simulink model "mavsim_L_t"  (R2023b)
settings: Solver=ode45  StartTime=0.0  StopTime=40  RelTol=1e-3  EnableMultiTasking=on
values from neighbouring files (symbols this model uses):
  P = (eye(17) - L*H)*P    [Estimator.m]
undefined symbols (not defined in the file or in its folder): barometer, drawAircraft_v2, Euler_to_Ra2b, forces_moments, gps, plotmavstatevariables, POS_smoother2, Pressure2Altitude
libraries: simulink x4, spsStairGeneratorLib x3, shared6dof x1, aerolibnav x1
settings Model: Creator=beard  LastModifiedBy=13995
settings SolverCC: AlgebraicLoopSolver=TrustRegion
settings DataIOCC: SaveFormat=Array
settings OptimizationCC: ExpressionDepthLimit=2147483647  InitFltsAndDblsToZero=on  LifeSpan=inf
settings DebuggingCC: UnderspecifiedInitializationDetection=Classic  MergeDetectMultiDrivingBlocksExec=none  SolverPrmCheckMsg=warning  UnconnectedInputMsg=warning  UnconnectedOutputMsg=warning  UnconnectedLineMsg=warning  StateNameClashWarn=warning  SFUnexpectedBacktrackingDiag=warning  SFNoUnconditionalDefaultTransitionDiag=warning  SFExecutionAtInitializationDiag=none  ArithmeticOperatorsInVariantConditions=warning
settings HardwareCC: ProdBitPerPointer=32  ProdBitPerSizeT=32  ProdBitPerPtrDiffT=32  ProdLargestAtomicFloat=None  ProdIntDivRoundTo=Undefined  ProdEndianess=Unspecified  ProdWordSize=32  ProdHWDeviceType=32-bit Generic
settings ModelReferenceCC: EnableRefExpFcnMdlSchedulingChecks=on  PropagateSignalLabelsOutOfModel=off
settings SFSimCC: SimUseLocalCustomCode=off  CustomCodeUndefinedFunction=UseInterfaceOnly
settings RTWCC: RTWUseLocalCustomCode=off
settings CodeAppCC: StateflowObjectComments=on
settings GRTTargetCC: TargetLangStandard=C89/C90 (ANSI)  CombineOutputUpdateFcns=off  GRTInterface=on
settings ConfigComp: CovMetricSettings=dw  CovSaveCumulativeToWorkspaceVar=on  CovSaveSingleToWorkspaceVar=on  CovExternalEMLEnable=off  CovSFcnEnable=off
settings SimscapeCC: SimscapeNormalizeSystem=off

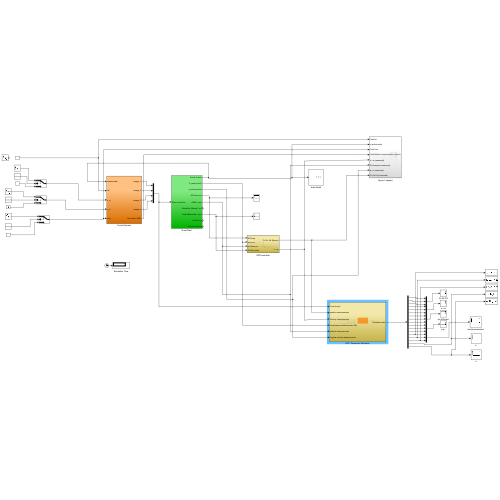
[thumbnail: Simulink's stored preview of the top-level diagram]
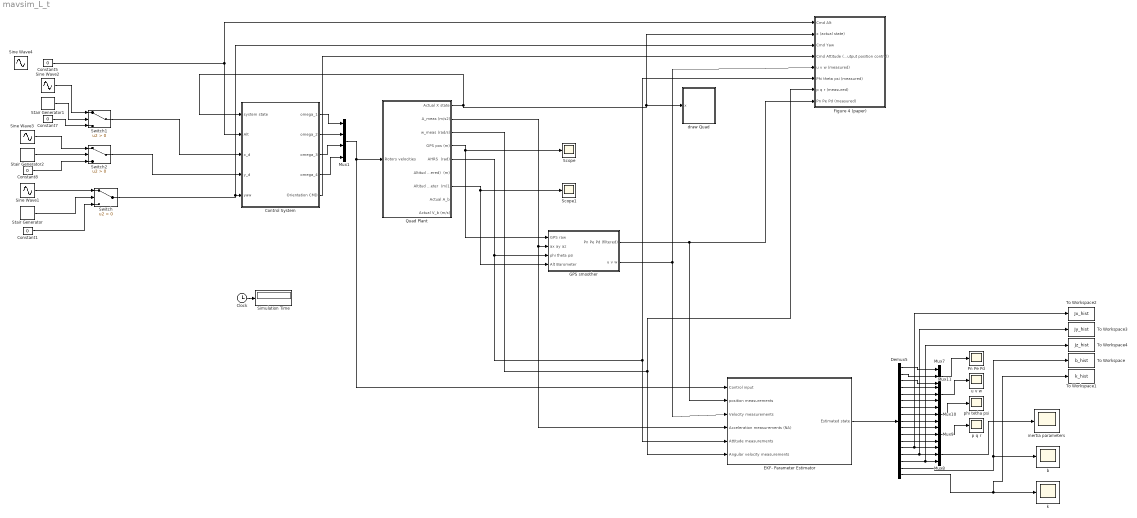
== system mavsim_L_t ==
  Clock : Clock
  Constant{1,5,7..8} (4 alike) : Constant  Value=0
  Control System : Subsystem
  Demux5 : Demux  Outputs=17
  EKF- Parameter Estimator : Subsystem
  Figure 4 (paper) : Subsystem
  GPS smoother : Subsystem
  Mux1 : Mux
  Mux{7..11} (5 alike) : Mux  Inputs=3
  Pn Pe Pd : Scope
  Quad Plant : Subsystem
  Scope : Scope
  Scope1 : Scope
  Simulation Time : Display
  Sine Wave1 : Sin  Amplitude=.45  Frequency=1.5  SampleTime=0
  Sine Wave2 : Sin  Frequency=2  SampleTime=0
  Sine Wave3 : Sin  Frequency=2  Phase=pi/2  SampleTime=0
  Sine Wave4 : Sin  Frequency=2  SampleTime=0
  Stair Generator : spsStairGeneratorLib/Stair Generator  t=[0, 5, 10, 15, 20, 25, 30 ,35,40]  e=[1, 1,1, 1,1,1,1,1,1]  Ts=0
  Stair Generator1 : spsStairGeneratorLib/Stair Generator  t=[0, 5, 10, 15, 20, 25, 30 ,35]  e="[1, 1,  1, 1, 1, 1, 1, 1]"  Ts=0
  Stair Generator2 : spsStairGeneratorLib/Stair Generator  t=[0, 5, 10, 15, 20, 25, 30 ,35]  e="[1, 1, 1 , 1, 1, 1, 1,  1]"  Ts=0
  Switch : Switch  Criteria=u2 > Threshold  SaturateOnIntegerOverflow=off  InputSameDT=off
  Switch1 : Switch  Criteria=u2 > Threshold  SaturateOnIntegerOverflow=off  InputSameDT=off
  Switch2 : Switch  Criteria=u2 > Threshold  SaturateOnIntegerOverflow=off  InputSameDT=off
  To Workspace : ToWorkspace  VariableName=b_hist  SaveFormat=Timeseries  SampleTime=-1
  To Workspace1 : ToWorkspace  VariableName=k_hist  SaveFormat=Timeseries  SampleTime=-1
  To Workspace2 : ToWorkspace  VariableName=Jx_hist  SaveFormat=Timeseries  SampleTime=-1
  To Workspace3 : ToWorkspace  VariableName=Jy_hist  SaveFormat=Timeseries  SampleTime=-1
  To Workspace4 : ToWorkspace  VariableName=Jz_hist  SaveFormat=Timeseries  SampleTime=-1
  b : Scope
  draw Quad : Subsystem
      mask init:
      | % parameters for drawing aircraft
      |   % scale size
      |   size = 20;
      |   fuse_l1    = 7;
      |   fuse_l2    = 4;
      |   fuse_l3    = 15;
      |   fuse_w     = 2;
      |   wing_l     = 6;
      |   wing_w     = 20;
      |   tail_l     = 3;
      |   tail_h     = 3;
      |   tailwing_w = 10;
      |   tailwing_l = 3;
      |   % colors
      |   red     = [1, 0, 0];
      |   green   = [0, 1, 0];
      |   blue    = [0, 0, 1];
      |   yellow  = [1,1,0];
      |   magenta = [0, 1, 1];
      |   
      | 
      | % define vertices and faces for aircraft
      |   V = [...
      |     fuse_l1,             0,             0;...        % point 1
      |     fuse_l2,            -fuse_w/2,     -fuse_w/2;... % point 2     
      |     fuse_l2,             fuse_w/2,     -fuse_w/2;... % point 3     
      |     fuse_l2,             fuse_w/2,      fuse_w/2;... % point 4
      |     fuse_l2,            -fuse_w/2,      fuse_w/2;... % point 5
      |    -fuse_l3,             0,             0;...        % point 6
      |     0,                   wing_w/2,      0;...        % point 7
      |    -wing_l,              wing_w/2,      0;...        % point 8
      |    -wing_l,             -wing_w/2,      0;...        % point 9
      |     0,                  -wing_w/2,      0;...        % point 10
      |    -fuse_l3+tailwing_l,  tailwing_w/2,  0;...        % point 11
      |    -fuse_l3,             tailwing_w/2,  0;...        % point 12
      |    -fuse_l3,            -tailwing_w/2,  0;...        % point 13
      |    -fuse_l3+tailwing_l, -tailwing_w/2,  0;...        % point 14
      |    -fuse_l3+tailwing_l,  0,             0;...        % point 15
      |    -fuse_l3+tailwing_l,  0,             -tail_h;...  % point 16
      |    -fuse_l3,             0,             -tail_h;...  % point 17
      |   ];
      |   
      |   F = [...
      |         1,  2,  3,  1;... % nose-top
      |         1,  3,  4,  1;... % nose-left
      |         1,  4,  5,  1;... % nose-bottom
      |         1,  5,  2,  1;... % nose-right
      |         2,  3,  6,  2;... % fuselage-top
      |         3,  6,  4,  3;... % fuselage-left
      |         4,  6,  5,  4;... % fuselage-bottom
      |         2,  5,  6,  2;... % fuselage-right
      |         7,  8,  9, 10;... % wing
      |        11, 12, 13, 14;... % tailwing
      |         6, 15, 17, 17;... % tail
      |         
      |   ];  
      |   
      |   colors = [...
      |         yellow;... % nose-top
      |         yellow;... % nose-left
      |         yellow;... % nose-bottom
      |         yellow;... % nose-right
      |         blue;... % fuselage-top
      |         blue;... % fuselage-left
      |         red;... % fuselage-bottom
      |         blue;... % fuselage-right
      |         green;... % wing
      |         green;... % tailwing
      |         blue;... % tail
      |     ];
      | 
      |   V = size*V;   % rescale vertices
      mask Display: image('tv.jpg')
  inertia parameters : Scope
  k : Scope
  p q r : Scope
  phi tetha psi : Scope
  u v w : Scope
  wires:
  Clock/1 -> Simulation Time/1
  Control System/1(omega_1) -> Mux1/1
  Control System/2(omega_2) -> Mux1/2
  Control System/3(omega_3) -> Mux1/3
  Control System/4(omega_4) -> Mux1/4
  Quad Plant/1(Actual X state) -> Figure 4 (paper)/2(x (actual state)), draw Quad/1(x), Control System/1("system state ")
  Mux1/1 -> EKF- Parameter Estimator/1(Control input), Quad Plant/1(Rotors velocities)
  Quad Plant/2(A_meas (m/s2)) -> EKF- Parameter Estimator/4(Acceleration measurements (NA)), GPS smoother/2(ax ay az)
  Quad Plant/3(w_meas (rad/s)) -> EKF- Parameter Estimator/6(Angular velocity measurements), Figure 4 (paper)/7(p q r (measured))
  Quad Plant/5(AHRS  (rad)) -> GPS smoother/3(phi theta psi), EKF- Parameter Estimator/5(Attitude measurements), Figure 4 (paper)/6(Phi theta psi (measured))
  Demux5/1 -> Mux7/1
  Demux5/2 -> Mux7/2
  Demux5/3 -> Mux7/3
  Mux7/1 -> Pn Pe Pd/1
  Demux5/13 -> To Workspace2/1, Mux8/1
  Demux5/14 -> To Workspace3/1, Mux8/2
  Demux5/15 -> To Workspace4/1, Mux8/3
  Mux8/1 -> inertia parameters/1
  Demux5/16 -> To Workspace/1, b/1
  Demux5/17 -> To Workspace1/1, k/1
  Demux5/12 -> Mux9/3
  Demux5/11 -> Mux9/2
  Demux5/10 -> Mux9/1
  Mux9/1 -> p q r/1
  Demux5/7 -> Mux10/1
  Demux5/8 -> Mux10/2
  Demux5/9 -> Mux10/3
  Mux10/1 -> phi tetha psi/1
  Demux5/4 -> Mux11/1
  Demux5/5 -> Mux11/2
  Demux5/6 -> Mux11/3
  Mux11/1 -> u v w/1
  Constant5/1 -> Figure 4 (paper)/1(Cmd Alt), Control System/2(Alt)
  Switch/1 -> Figure 4 (paper)/3(Cmd Yaw), Control System/5(yaw)
  Sine Wave1/1 -> Switch/1
  Constant1/1 -> Switch/3
  Stair Generator/1 -> Switch/2
  Switch1/1 -> Control System/3(x_d)
  Stair Generator1/1 -> Switch1/2
  Sine Wave2/1 -> Switch1/1
  Constant7/1 -> Switch1/3
  Switch2/1 -> Control System/4(y_d)
  Stair Generator2/1 -> Switch2/2
  Sine Wave3/1 -> Switch2/1
  Constant8/1 -> Switch2/3
  Control System/5(Orientation CMD) -> Figure 4 (paper)/4(Cmd Attitude (output position control))
  EKF- Parameter Estimator/1(Estimated state) -> Demux5/1
  GPS smoother/2(u v w) -> Figure 4 (paper)/5(u v w (measured)), EKF- Parameter Estimator/3(Velocity measurements)
  GPS smoother/1(Pn Pe Pd (filtered)) -> Figure 4 (paper)/8(Pn Pe Pd (measured)), EKF- Parameter Estimator/2(position measurements)
  Quad Plant/4(GPS pos (m)) -> Scope/1, GPS smoother/1(GPS raw)
  Quad Plant/7(Altitud Barometer  (m)1) -> Scope1/1, GPS smoother/4(Alt Barometer)

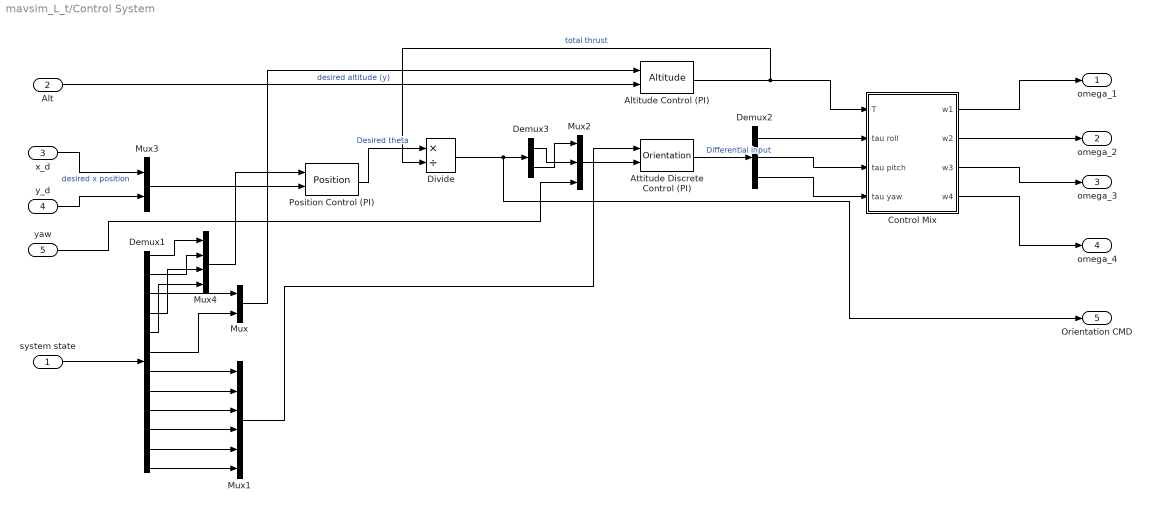
== system mavsim_L_t/Control System ==
  "system state " : Inport
  Alt : Inport  Port=2
  x_d : Inport  Port=3
  y_d : Inport  Port=4
  yaw : Inport  Port=5
  Altitude Control (PI) : M-S-Function  FunctionName=Altitude  Parameters=P
  Attitude Discrete Control (PI) : M-S-Function  FunctionName=Orientation  Parameters=P
  Control Mix : Subsystem
  Demux1 : Demux  Outputs=12
  Demux2 : Demux  Outputs=3
  Demux3 : Demux  Outputs=2
  Divide : Product  Inputs=*/
  Mux : Mux  Inputs=2
  Mux1 : Mux  Inputs=6
  Mux2 : Mux  Inputs=3
  Mux3 : Mux  Inputs=2
  Mux4 : Mux
  Position Control (PI) : M-S-Function  FunctionName=Position  Parameters=P
  omega_1 : Outport  VectorParamsAs1DForOutWhenUnconnected=off
  omega_2 : Outport  Port=2  VectorParamsAs1DForOutWhenUnconnected=off
  omega_3 : Outport  Port=3  VectorParamsAs1DForOutWhenUnconnected=off
  omega_4 : Outport  Port=4  VectorParamsAs1DForOutWhenUnconnected=off
  Orientation CMD : Outport  Port=5  VectorParamsAs1DForOutWhenUnconnected=off
  wires:
  Alt/1 -> Altitude Control (PI)/2  "desired altitude (y)"
  Control Mix/1(w1) -> omega_1/1
  Control Mix/2(w2) -> omega_2/1
  Control Mix/3(w3) -> omega_3/1
  Control Mix/4(w4) -> omega_4/1
  Demux1/3 -> Mux/1
  Demux1/6 -> Mux/2
  Mux/1 -> Altitude Control (PI)/1
  Altitude Control (PI)/1 -> Divide/2, Control Mix/1(T)  "total thrust"
  "system state "/1 -> Demux1/1
  Demux1/7 -> Mux1/1
  Demux1/8 -> Mux1/2
  Demux1/9 -> Mux1/3
  Demux1/10 -> Mux1/4
  Demux1/11 -> Mux1/5
  Demux1/12 -> Mux1/6
  Mux1/1 -> Attitude Discrete Control (PI)/1
  Mux2/1 -> Attitude Discrete Control (PI)/2
  Attitude Discrete Control (PI)/1 -> Demux2/1  "Differential input"
  Demux2/1 -> Control Mix/2(tau roll)
  Demux2/2 -> Control Mix/3(tau pitch)
  Demux2/3 -> Control Mix/4(tau yaw)
  x_d/1 -> Mux3/1  "desired x position"
  y_d/1 -> Mux3/2
  Mux3/1 -> Position Control (PI)/2
  Demux1/1 -> Mux4/1
  Demux1/2 -> Mux4/2
  Demux1/4 -> Mux4/3
  Demux1/5 -> Mux4/4
  Mux4/1 -> Position Control (PI)/1
  Position Control (PI)/1 -> Divide/1  "Desired theta"
  yaw/1 -> Mux2/3
  Demux3/2 -> Mux2/1
  Divide/1 -> Orientation CMD/1, Demux3/1
  Demux3/1 -> Mux2/2

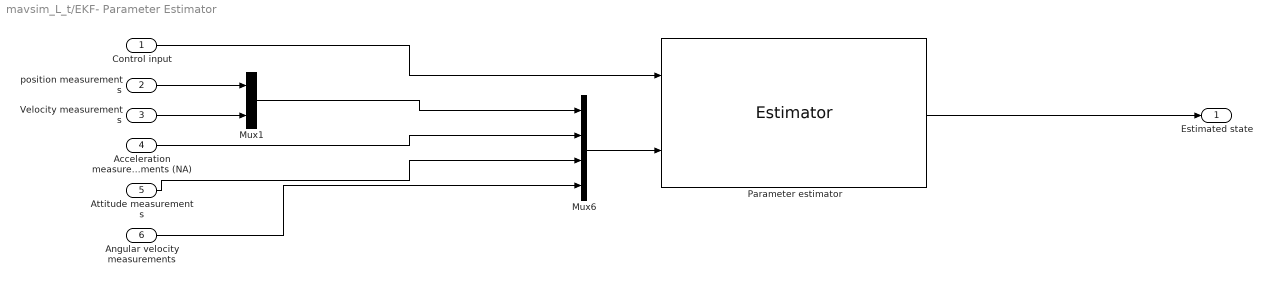
== system mavsim_L_t/EKF- Parameter Estimator ==
  Control input : Inport
  position measurements : Inport  Port=2
  Velocity measurements : Inport  Port=3
  Acceleration measurements (NA) : Inport  Port=4
  Attitude measurements : Inport  Port=5
  Angular velocity measurements : Inport  Port=6
  Mux1 : Mux  Inputs=2
  Mux6 : Mux
  "Parameter estimator " : M-S-Function  FunctionName=Estimator  Parameters=P
  Estimated state : Outport
  wires:
  Control input/1 -> "Parameter estimator "/1
  Attitude measurements/1 -> Mux6/3
  Acceleration measurements (NA)/1 -> Mux6/2
  Mux6/1 -> "Parameter estimator "/2
  "Parameter estimator "/1 -> Estimated state/1
  Angular velocity measurements/1 -> Mux6/4
  Mux1/1 -> Mux6/1
  position measurements/1 -> Mux1/1
  Velocity measurements/1 -> Mux1/2

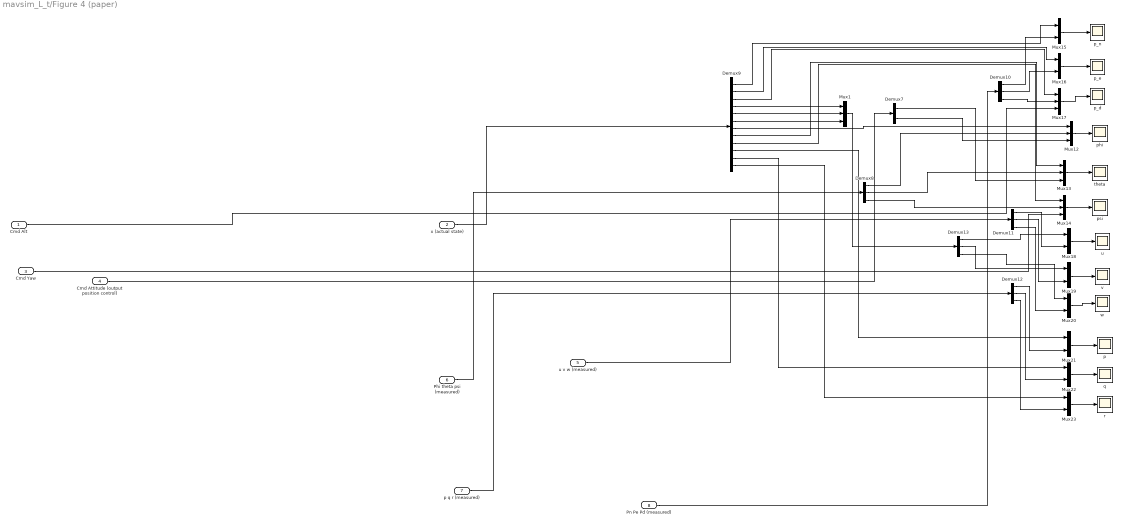
== system mavsim_L_t/Figure 4 (paper) ==
  Cmd Alt : Inport
  x (actual state) : Inport  Port=2
  Cmd Yaw : Inport  Port=3
  Cmd Attitude (output position control) : Inport  Port=4
  u v w (measured) : Inport  Port=5
  Phi theta psi (measured) : Inport  Port=6
  p q r (measured) : Inport  Port=7
  Pn Pe Pd (measured) : Inport  Port=8
  Demux{8,10..13} (5 alike) : Demux  Outputs=3
  Demux7 : Demux  Outputs=2
  Demux9 : Demux  Outputs=12
  Mux{1,12..14,17} (5 alike) : Mux  Inputs=3
  Mux{15..16,18..23} (8 alike) : Mux  Inputs=2
  p : Scope
  p_d : Scope
  p_e : Scope
  p_n : Scope
  phi : Scope
  psi : Scope
  q : Scope
  r : Scope
  theta : Scope
  u : Scope
  v : Scope
  w : Scope
  wires:
  Mux12/1 -> phi/1
  Demux8/3 -> Mux14/2
  Mux21/1 -> p/1
  p q r (measured)/1 -> Demux12/1
  Mux20/1 -> w/1
  Demux9/8 -> Mux13/1
  u v w (measured)/1 -> Demux11/1
  Demux9/11 -> Mux22/1
  Mux13/1 -> theta/1
  Demux11/1 -> Mux18/2
  Mux18/1 -> u/1
  Demux8/2 -> Mux13/2
  Demux9/7 -> Mux12/1
  Phi theta psi (measured)/1 -> Demux8/1
  Demux9/6 -> Mux1/3
  x (actual state)/1 -> Demux9/1
  Cmd Yaw/1 -> Mux14/3
  Demux9/10 -> Mux21/1
  Mux14/1 -> psi/1
  Demux9/12 -> Mux23/1
  Demux10/1 -> Mux15/2
  Demux10/2 -> Mux16/2
  Demux9/2 -> Mux16/1
  Demux12/3 -> Mux23/2
  Demux10/3 -> Mux17/2
  Mux17/1 -> p_d/1
  Mux19/1 -> v/1
  Demux9/1 -> Mux15/1
  Demux9/5 -> Mux1/2
  Demux8/1 -> Mux12/2
  Demux12/2 -> Mux22/2
  Cmd Alt/1 -> Mux17/3
  Demux13/1 -> Mux18/1
  Mux16/1 -> p_e/1
  Cmd Attitude (output position control)/1 -> Demux7/1
  Demux7/1 -> Mux13/3
  Mux15/1 -> p_n/1
  Demux11/3 -> Mux20/2
  Demux7/2 -> Mux12/3
  Demux12/1 -> Mux21/2
  Demux13/2 -> Mux19/1
  Mux23/1 -> r/1
  Demux9/3 -> Mux17/1
  Demux9/9 -> Mux14/1
  Pn Pe Pd (measured)/1 -> Demux10/1
  Demux11/2 -> Mux19/2
  Demux13/3 -> Mux20/1
  Demux9/4 -> Mux1/1
  Mux22/1 -> q/1
  Mux1/1 -> Demux13/1

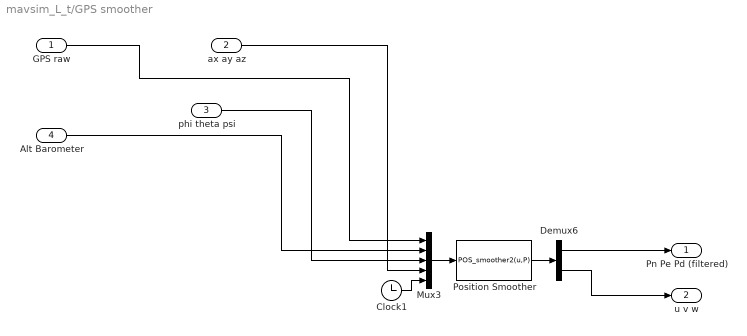
== system mavsim_L_t/GPS smoother ==
  GPS raw : Inport
  ax ay az : Inport  Port=2
  phi theta psi : Inport  Port=3
  Alt Barometer : Inport  Port=4
  Clock1 : Clock
  Demux6 : Demux  Outputs=2
  Mux3 : Mux  Inputs=5
  "Position Smoother " : MATLABFcn  MATLABFcn=POS_smoother2(u,P)  OutputDimensions=6  SampleTime=P.GPSsm.dt
  Pn Pe Pd (filtered) : Outport
  u v w : Outport  Port=2
  wires:
  Clock1/1 -> Mux3/5
  Demux6/1 -> Pn Pe Pd (filtered)/1
  Alt Barometer/1 -> Mux3/2
  phi theta psi/1 -> Mux3/3
  Demux6/2 -> u v w/1
  ax ay az/1 -> Mux3/4
  "Position Smoother "/1 -> Demux6/1
  GPS raw/1 -> Mux3/1
  Mux3/1 -> "Position Smoother "/1

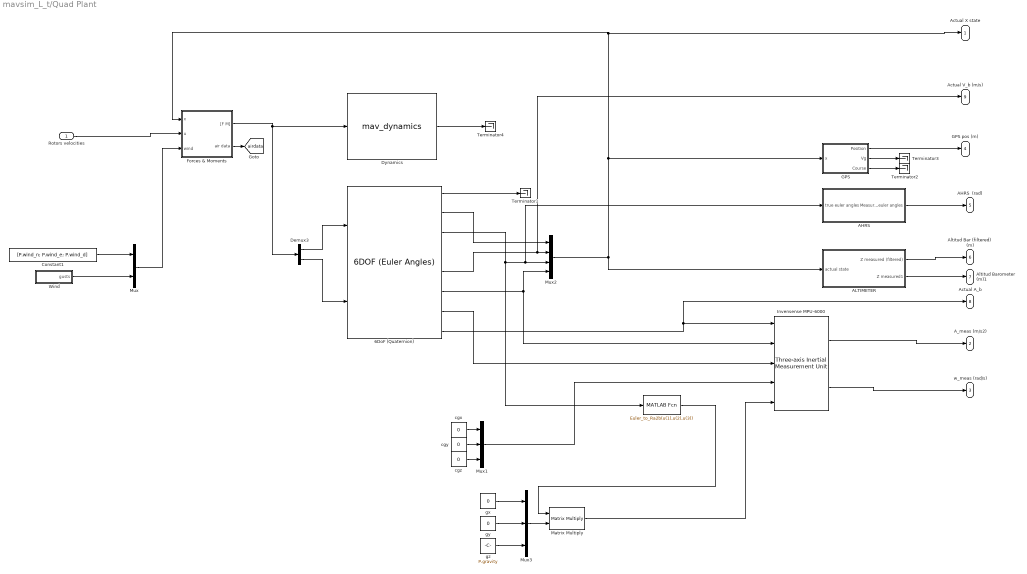
== system mavsim_L_t/Quad Plant ==
  Rotors velocities : Inport
  " " : MATLABFcn  MATLABFcn=Euler_to_Ra2b(u(1),u(2),u(3))  OutputDimensions=[3 3]  Output1D=off
  6DoF (Quaternion) : shared6dof/6DOF (Euler Angles)  units=Metric (MKS)  mtype=Fixed  rep=Quaternion  xme_0=[0 0 0]  Vm_0=[0 0 0]  eul_0=[0 0 0]  pm_0=[0 0 0]  mass_0=P.mass  mass_e=0  mass_f=0  inertia=[P.Jx, 0, 0; 0, P.Jy, 0; 0, 0, P.Jz]  inertia_e=eye(3)  inertia_f=eye(3)  k_quat=1.0  vre_flag=on  abi_flag=off  aMode=0  xme_statename=''  Vm_statename=''  eul_statename=''  quat_statename=''  pm_statename=''  mass_statename=''
  AHRS : Subsystem
  ALTIMETER : Subsystem
  Constant1 : Constant  Value=[P.wind_n; P.wind_e; P.wind_d]
  Demux3 : Demux  Outputs=2
  Dynamics : S-Function  FunctionName=mav_dynamics  Parameters=mass,Jx,Jy,Jz,Jxz,pn0,pe0,pd0,u0,v0,w0,phi0,theta0,psi0,p0,q0,r0  SFunctionDeploymentMode=off  EnableBusSupport=off  mask{mass=P.mass, Jx=P.Jx, Jy=P.Jy, Jz=P.Jz, Jxz=P.Jxz, pn0=P.pn0, pe0=P.pe0, pd0=P.pd0, u0=P.u0, v0=P.v0, w0=P.w0, phi0=P.phi0, theta0=P.theta0, psi0=P.psi0, p0=P.p0, q0=P.q0, r0=P.r0}
      mask prompts: pn0 "Initial North position"; pe0 "Initial East position"; pd0 "Initial Down position"; u0 "Initial velocy u0"; v0 "Initial velocity v0"; w0 "Initial velocity w0"; phi0 "Initial roll angle"; theta0 "Initial pitch angle"; psi0 "Initial yaw angle"; p0 "Initial roll rate"; q0 "Initial pitch rate"; r0 "Initial yaw rate"
  Forces & Moments : Subsystem
  GPS : Subsystem
  Invensense MPU-6000 : aerolibnav/Three-axis Inertial Measurement Unit  units=Metric (MKS)  imu=[0 0 0]  i_Ts=0.004  dtype_a=off  w_a=190  z_a=0.707  a_sf_cc=[0.98 0 0; 0 0.98 0; 0 0 0.98]  a_bias=P.IMUAccel_bias  a_sat="[-19.62  -19.62  -19.62 19.62 19.62 19.62]"  dtype_g=off  w_g=190  z_g=0.707  g_sf_cc=[.98 0 0; 0 .98 0; 0 0 .98]  g_bias=[0 0 0]  g_sens=[0 0 0]  g_sat="[-4.36  -4.36  -4.36 4.36 4.36 4.36]"  i_rand=on  i_seeds=[348631 366719 978432 189621 128794 214632]  i_pow=P.IMUnoise
  Matrix Multiply : Product  Multiplication=Matrix(*)
  Mux : Mux  Inputs=2
  Mux1 : Mux  Inputs=3
  Mux2 : Mux
  Mux3 : Mux  Inputs=3
  Terminator{1..4} (4 alike) : Terminator
  Wind : Subsystem
  cgx : Constant  Value=0
  cgy : Constant  Value=0
  cgz : Constant  Value=0
  gx : Constant  Value=0
  gy : Constant  Value=0
  gz : Constant  Value=P.gravity
  Actual X state : Outport  VectorParamsAs1DForOutWhenUnconnected=off
  A_meas (m/s2) : Outport  Port=2  VectorParamsAs1DForOutWhenUnconnected=off
  w_meas (rad/s) : Outport  Port=3  VectorParamsAs1DForOutWhenUnconnected=off
  GPS pos (m) : Outport  Port=4  VectorParamsAs1DForOutWhenUnconnected=off
  AHRS  (rad) : Outport  Port=5  VectorParamsAs1DForOutWhenUnconnected=off
  Altitud Bar (filtered)  (m) : Outport  Port=6  VectorParamsAs1DForOutWhenUnconnected=off
  Altitud Barometer  (m)1 : Outport  Port=7  VectorParamsAs1DForOutWhenUnconnected=off
  Actual A_b : Outport  Port=8  VectorParamsAs1DForOutWhenUnconnected=off
  Actual V_b (m/s) : Outport  Port=9  VectorParamsAs1DForOutWhenUnconnected=off
  tag scope: airdata=global
  wires:
  6DoF (Quaternion)/2 -> Mux2/1
  Demux3/2 -> 6DoF (Quaternion)/2
  6DoF (Quaternion)/3 -> " "/1, AHRS/1(true euler angles), Mux2/3
  6DoF (Quaternion)/6 -> Invensense MPU-6000/2, Mux2/4
  Mux2/1 -> ALTIMETER/1(actual state), GPS/1(x), Actual X state/1, Forces & Moments/1(x)
  Demux3/1 -> 6DoF (Quaternion)/1
  Forces & Moments/1("[F M]") -> Demux3/1, Dynamics/1
  Mux/1 -> Forces & Moments/3(wind)
  Wind/1(gusts) -> Mux/2
  Constant1/1 -> Mux/1
  Forces & Moments/2(air data) -> [airdata]
  Rotors velocities/1 -> Forces & Moments/2(u)
  Dynamics/1 -> Terminator4/1
  6DoF (Quaternion)/1 -> Terminator1/1
  6DoF (Quaternion)/5 -> Actual V_b (m/s)/1, Mux2/2
  6DoF (Quaternion)/7 -> Invensense MPU-6000/3
  cgz/1 -> Mux1/3
  cgx/1 -> Mux1/1
  cgy/1 -> Mux1/2
  Mux1/1 -> Invensense MPU-6000/4
  Mux3/1 -> Matrix Multiply/2
  gz/1 -> Mux3/3
  gx/1 -> Mux3/1
  gy/1 -> Mux3/2
  Invensense MPU-6000/2 -> w_meas (rad/s)/1
  GPS/3(Course) -> Terminator2/1
  GPS/2(Vg) -> Terminator3/1
  GPS/1(Position) -> GPS pos (m)/1
  AHRS/1(Measured euler angles) -> AHRS  (rad)/1
  ALTIMETER/1(Z measured (filtered)) -> Altitud Bar (filtered)  (m)/1
  ALTIMETER/2(Z measured1) -> Altitud Barometer  (m)1/1
  6DoF (Quaternion)/8 -> Actual A_b/1, Invensense MPU-6000/1
  Invensense MPU-6000/1 -> A_meas (m/s2)/1
  " "/1 -> Matrix Multiply/1
  Matrix Multiply/1 -> Invensense MPU-6000/5

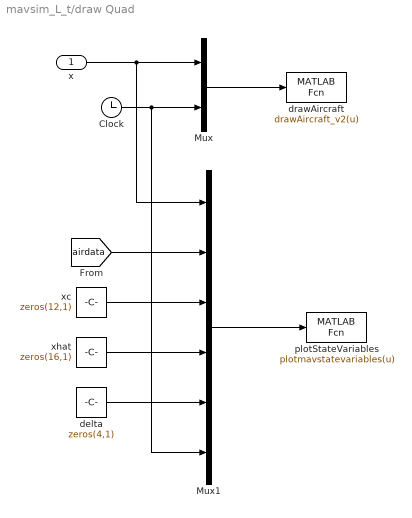
== system mavsim_L_t/draw Quad ==
  x : Inport
  Clock : Clock
  Mux : Mux  Inputs=2
  Mux1 : Mux  Inputs=6
  delta : Constant  Value=zeros(4,1)
  drawAircraft : MATLABFcn  MATLABFcn=drawAircraft_v2(u)  OutputDimensions=0  SampleTime=0.1
  plotStateVariables : MATLABFcn  MATLABFcn=plotmavstatevariables(u)  OutputDimensions=0  SampleTime=0.1
  xc : Constant  Value=zeros(12,1)
  xhat : Constant  Value=zeros(16,1)
  wires:
  [airdata] -> Mux1/2
  delta/1 -> Mux1/5
  xc/1 -> Mux1/3
  xhat/1 -> Mux1/4
  Mux1/1 -> plotStateVariables/1
  Clock/1 -> Mux1/6, Mux/2
  x/1 -> Mux1/1, Mux/1
  Mux/1 -> drawAircraft/1

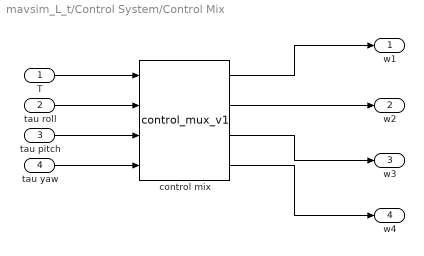
== system mavsim_L_t/Control System/Control Mix ==
  T : Inport
  tau roll : Inport  Port=2
  tau pitch : Inport  Port=3
  tau yaw : Inport  Port=4
  control mix : M-S-Function  FunctionName=control_mux_v1
  w1 : Outport  VectorParamsAs1DForOutWhenUnconnected=off
  w2 : Outport  Port=2  VectorParamsAs1DForOutWhenUnconnected=off
  w3 : Outport  Port=3  VectorParamsAs1DForOutWhenUnconnected=off
  w4 : Outport  Port=4  VectorParamsAs1DForOutWhenUnconnected=off
  wires:
  control mix/2 -> w2/1
  T/1 -> control mix/1
  tau roll/1 -> control mix/2
  tau pitch/1 -> control mix/3
  tau yaw/1 -> control mix/4
  control mix/4 -> w4/1
  control mix/3 -> w3/1
  control mix/1 -> w1/1

== system mavsim_L_t/Quad Plant/AHRS ==
  true euler angles : Inport
  Band-Limited White Noise : simulink/Sources/Band-Limited White Noise  Cov=P.zAttNoise  Ts=0.1  seed=[23341]
  Sum : Sum  Inputs=|++  SampleTime=P.Ts_AHRS
  Measured euler angles : Outport  VectorParamsAs1DForOutWhenUnconnected=off
  wires:
  Sum/1 -> Measured euler angles/1
  true euler angles/1 -> Sum/1
  Band-Limited White Noise/1 -> Sum/2

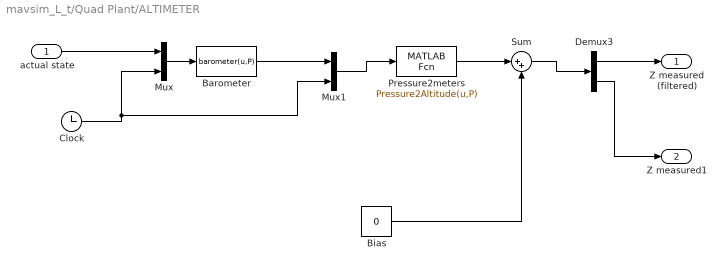
== system mavsim_L_t/Quad Plant/ALTIMETER ==
  actual state : Inport
  Barometer : MATLABFcn  MATLABFcn=barometer(u,P)  OutputDimensions=1  SampleTime=P.Ts_Barometer
  Bias : Constant  Value=0
  Clock : Clock
  Demux3 : Demux  Outputs=2
  Mux : Mux  Inputs=2
  Mux1 : Mux  Inputs=2
  Pressure2meters : MATLABFcn  MATLABFcn=Pressure2Altitude(u,P)  OutputDimensions=2  SampleTime=P.Ts_Barometer
  Sum : Sum  Inputs=|++
  Z measured (filtered) : Outport  VectorParamsAs1DForOutWhenUnconnected=off
  Z measured1 : Outport  Port=2  VectorParamsAs1DForOutWhenUnconnected=off
  wires:
  Clock/1 -> Mux1/2, Mux/2
  Mux/1 -> Barometer/1
  Barometer/1 -> Mux1/1
  Mux1/1 -> Pressure2meters/1
  Pressure2meters/1 -> Sum/1
  Bias/1 -> Sum/2
  actual state/1 -> Mux/1
  Sum/1 -> Demux3/1
  Demux3/1 -> Z measured (filtered)/1
  Demux3/2 -> Z measured1/1

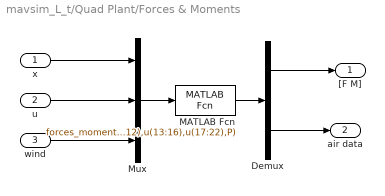
== system mavsim_L_t/Quad Plant/Forces & Moments ==
  x : Inport
  u : Inport  Port=2
  wind : Inport  Port=3
  Demux : Demux  Outputs=[6;6]
  MATLAB Fcn : MATLABFcn  MATLABFcn=forces_moments(u(1:12),u(13:16),u(17:22),P)  OutputDimensions=12
  Mux : Mux  Inputs=3
  "[F M]" : Outport  VectorParamsAs1DForOutWhenUnconnected=off
  air data : Outport  Port=2  VectorParamsAs1DForOutWhenUnconnected=off
  wires:
  x/1 -> Mux/1
  u/1 -> Mux/2
  wind/1 -> Mux/3
  MATLAB Fcn/1 -> Demux/1
  Demux/1 -> "[F M]"/1
  Mux/1 -> MATLAB Fcn/1
  Demux/2 -> air data/1

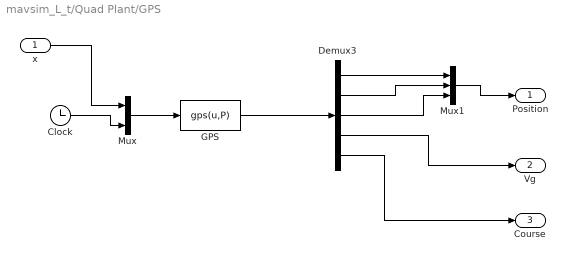
== system mavsim_L_t/Quad Plant/GPS ==
  x : Inport
  Clock : Clock
  Demux3 : Demux  Outputs=5
  GPS : MATLABFcn  MATLABFcn=gps(u,P)  OutputDimensions=5  SampleTime=P.Ts_gps
  Mux : Mux  Inputs=2
  Mux1 : Mux  Inputs=3
  Position : Outport  VectorParamsAs1DForOutWhenUnconnected=off
  Vg : Outport  Port=2  VectorParamsAs1DForOutWhenUnconnected=off
  Course : Outport  Port=3  VectorParamsAs1DForOutWhenUnconnected=off
  wires:
  x/1 -> Mux/1
  Clock/1 -> Mux/2
  Mux/1 -> GPS/1
  GPS/1 -> Demux3/1
  Demux3/1 -> Mux1/1
  Demux3/2 -> Mux1/2
  Demux3/3 -> Mux1/3
  Mux1/1 -> Position/1
  Demux3/4 -> Vg/1
  Demux3/5 -> Course/1

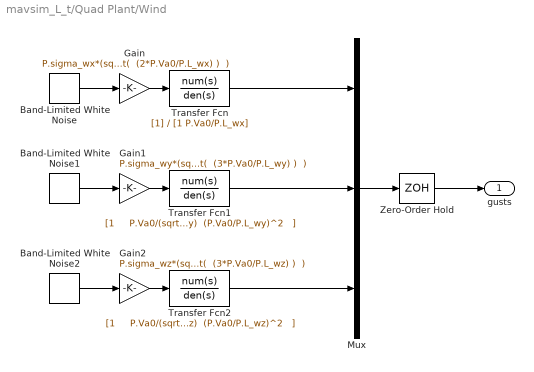
== system mavsim_L_t/Quad Plant/Wind ==
  Band-Limited White Noise : simulink/Sources/Band-Limited White Noise  Cov=[1]  Ts=0.1  seed=[23341]
  Band-Limited White Noise1 : simulink/Sources/Band-Limited White Noise  Cov=[1]  Ts=0.1  seed=[23541]
  Band-Limited White Noise2 : simulink/Sources/Band-Limited White Noise  Cov=[1]  Ts=0.1  seed=[21541]
  Gain : Gain  Gain="P.sigma_wx*(sqrt(  (2*P.Va0/P.L_wx) )  )"
  Gain1 : Gain  Gain="P.sigma_wy*(sqrt(  (3*P.Va0/P.L_wy) )  )"
  Gain2 : Gain  Gain="P.sigma_wz*(sqrt(  (3*P.Va0/P.L_wz) )  )"
  Mux : Mux  Inputs=3
  Transfer Fcn : TransferFcn  Denominator=[1 P.Va0/P.L_wx]
  Transfer Fcn1 : TransferFcn  Numerator="[1     P.Va0/(sqrt(3)*P.L_wy)]"  Denominator="[1     2*(P.Va0/P.L_wy)  (P.Va0/P.L_wy)^2   ]"
  Transfer Fcn2 : TransferFcn  Numerator="[1     P.Va0/(sqrt(3)*P.L_wz)]"  Denominator="[1     2*(P.Va0/P.L_wz)  (P.Va0/P.L_wz)^2   ]"
  Zero-Order Hold : ZeroOrderHold  SampleTime=P.Ts
  gusts : Outport  VectorParamsAs1DForOutWhenUnconnected=off
  wires:
  Transfer Fcn/1 -> Mux/1
  Transfer Fcn2/1 -> Mux/3
  Mux/1 -> Zero-Order Hold/1
  Zero-Order Hold/1 -> gusts/1
  Gain/1 -> Transfer Fcn/1
  Band-Limited White Noise/1 -> Gain/1
  Transfer Fcn1/1 -> Mux/2
  Gain1/1 -> Transfer Fcn1/1
  Band-Limited White Noise1/1 -> Gain1/1
  Gain2/1 -> Transfer Fcn2/1
  Band-Limited White Noise2/1 -> Gain2/1
